simulink model "NewApproach"  (R2022a)
settings: Solver=VariableStepAuto  StartTime=0.0  StopTime=43  FixedStep=0.05  RelTol=1e-3
undefined symbols (not defined in the file or in its folder): B, Spline, X, Y, Z
libraries: sm_lib x146, nesl_utility x22, fl_lib x6, sh_lib x3, robotcorelib x3, slpidlib x1
(part 1 of 5)
settings Model: Creator=Jakob  LastModifiedBy=Jakob

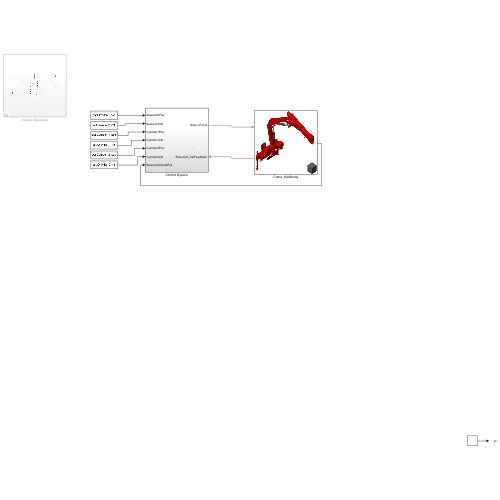
[thumbnail: Simulink's stored preview of the top-level diagram]
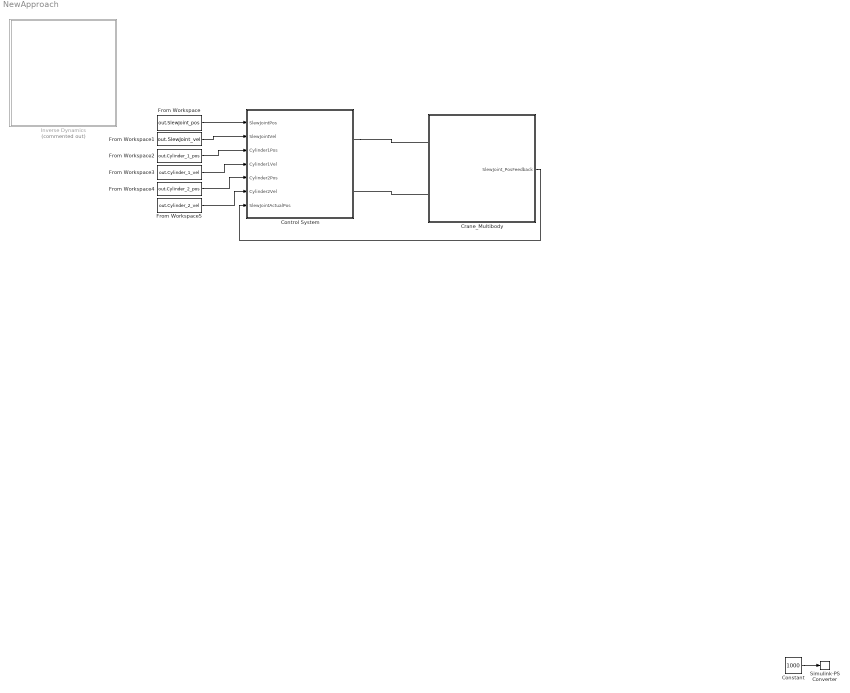
== system NewApproach ==
  Constant : Constant  Value=1000
  Control System : Subsystem
  Crane_Multibody : Subsystem
      mask Display: image('C:\Users\Jakob\OneDrive\Bilder\crane.PNG'); % Use "Edit Image" on toolstrip to change.
  From Workspace : FromWorkspace  VariableName=out.SlewJoint_pos
  From Workspace1 : FromWorkspace  VariableName=out.SlewJoint_vel
  From Workspace2 : FromWorkspace  VariableName=out.Cylinder_1_pos
  From Workspace3 : FromWorkspace  VariableName=out.Cylinder_1_vel
  From Workspace4 : FromWorkspace  VariableName=out.Cylinder_2_pos
  From Workspace5 : FromWorkspace  VariableName=out.Cylinder_2_vel
  Inverse Dynamics : Subsystem  Commented=on
  Simulink-PS Converter : nesl_utility/Simulink-PS Converter  PhysicalDomain=network_engine_domain  SubClassName=ps_input  LeftPortType=input  RightPortType=output  PseudoPeriodic=off  Frequencies=[]  NoiseDistribution=none  NoiseParameters=[]  Unit=1  AffineConversion=off  FilteringAndDerivatives=provide  SimscapeFilterOrder=1  InputFilterTimeConstant=0.001  UdotUserProvided=0
      settings: SourceProductBaseCode=SS,PW,VE
  wires:
  Constant/1 -> Simulink-PS Converter/1
  From Workspace5/1 -> Control System/6(Cylinder2Vel)
  From Workspace4/1 -> Control System/5(Cylinder2Pos)
  From Workspace3/1 -> Control System/4(Cylinder1Vel)
  From Workspace2/1 -> Control System/3(Cylinder1Pos)
  From Workspace1/1 -> Control System/2(SlewJointVel)
  From Workspace/1 -> Control System/1(SlewJointPos)
  Crane_Multibody/1(SlewJoint_PosFeedback) -> Control System/7(SlewJointActualPos)
  connections:
  Control System/RConn1 -- Crane_Multibody/LConn1
  Crane_Multibody/LConn2 -- Control System/RConn2

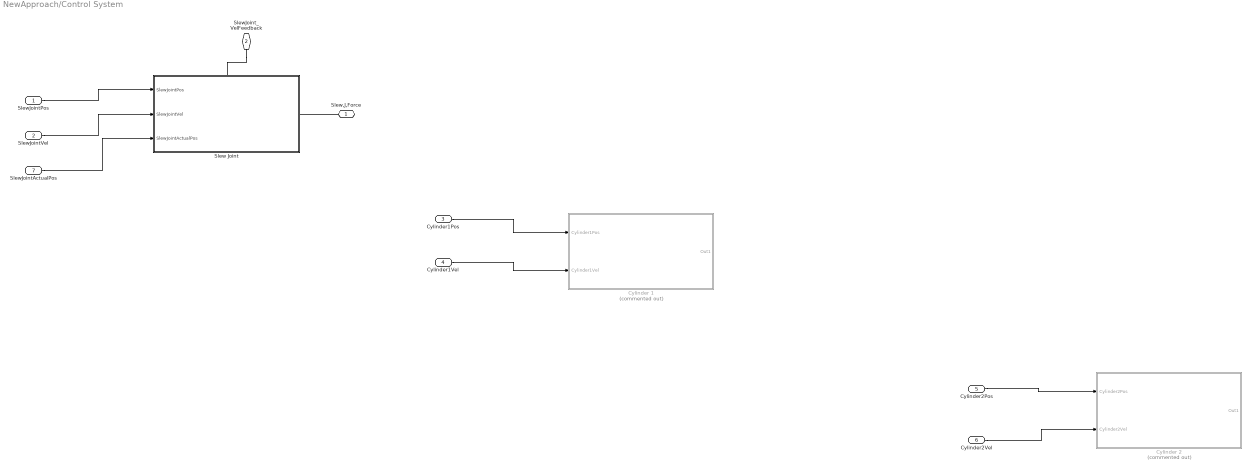
== system NewApproach/Control System ==
  SlewJointPos : Inport
  SlewJointVel : Inport  Port=2
  Cylinder1Pos : Inport  Port=3
  Cylinder1Vel : Inport  Port=4
  Cylinder2Pos : Inport  Port=5
  Cylinder2Vel : Inport  Port=6
  SlewJointActualPos : Inport  Port=7
  Cylinder 1 : Subsystem  Commented=on
  Cylinder 2 : Subsystem  Commented=on
  Slew Joint : Subsystem
      settings: PortSchema="{\"entries\":[{\"content\":{\"sides\":[{\"content\":{\"connectorIds\":[\"In1\",\"In2\",\"In3\"]},\"type\":\"ConnectorPlacement.EquallySpacedRectSide\",\"uuid\":\"c66543fa-198c-4f99-bad8-b3fba23087d9\"},{\"content\":{\"connectorIds\":[\"RConn1\"],\"side\":\"RIGHT\"},\"type\":\"ConnectorPlacement.EquallySpacedRectSide\",\"uuid\":\"68dc06a0-8d9d-4ec7-aacb-b23d2e6fbaba\"},{\"content\":{\"connectorIds\":[\"LConn1\"],\"side\":\"TOP\"},\"type\":\"ConnectorPlacement.EquallySpacedRectSide\",\"uuid\":\"7cecdc53-4657-4882-ad34-35515944277c\"}]},\"type\":\"ConnectorPlacement.EquallySpacedConnector\",\"uuid\":\"472e1db7-f81a-4c73-97d6-ba992d4f136f\"}],\"packageUris\":[\"http://schema.mathworks.com/mf0/Connector/R2020b\"],\"version\":\"1.0\"}"
  Slew,J,Force : PMIOPort  Side=Right
  SlewJoint_VelFeedback : PMIOPort  Port=2  Side=Right
  wires:
  Cylinder2Pos/1 -> Cylinder 2/1(Cylinder2Pos)
  Cylinder2Vel/1 -> Cylinder 2/2(Cylinder2Vel)
  Cylinder1Pos/1 -> Cylinder 1/1(Cylinder1Pos)
  Cylinder1Vel/1 -> Cylinder 1/2(Cylinder1Vel)
  SlewJointPos/1 -> Slew Joint/1(SlewJointPos)
  SlewJointVel/1 -> Slew Joint/2(SlewJointVel)
  SlewJointActualPos/1 -> Slew Joint/3(SlewJointActualPos)
  connections:
  Slew,J,Force/RConn1 -- Slew Joint/RConn1
  SlewJoint_VelFeedback/RConn1 -- Slew Joint/LConn1
